simulink model "week1_p3"  (R2020a)
settings: Solver=VariableStepAuto  StartTime=0.0  StopTime=10.0  RelTol=1e-3
settings Model: Creator=prabhudevmaddipudi  LastModifiedBy=prabhudevmaddipudi

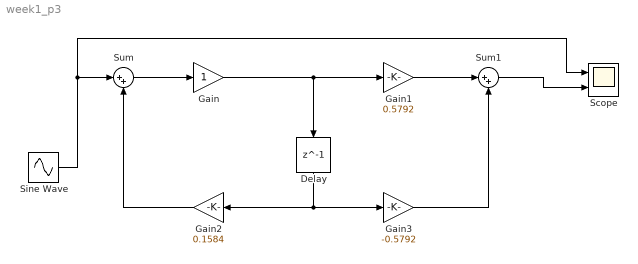
== system week1_p3 ==
  Delay : Delay  DelayLength=1
  Gain : Gain
  Gain1 : Gain  Gain=0.5792
  Gain2 : Gain  Gain=0.1584
  Gain3 : Gain  Gain=-0.5792
  Scope : Scope  NumInputPorts=2
  Sine Wave : Sin  Frequency=500  SampleTime=0
  Sum : Sum  Inputs=|++
  Sum1 : Sum  Inputs=|++
  wires:
  Delay/1 -> Gain3/1, Gain2/1
  Gain1/1 -> Sum1/1
  Sine Wave/1 -> Scope/1, Sum/1
  Sum1/1 -> Scope/2
  Gain/1 -> Delay/1, Gain1/1
  Gain2/1 -> Sum/2
  Sum/1 -> Gain/1
  Gain3/1 -> Sum1/2
